simulink model "ex_hb1ode"  (R2023a)
settings: Solver=ode15s  StartTime=0.0  StopTime=1e5
undefined symbols (not defined in the file): k1, k2, k3
settings Model: Creator=mosuk  LastModifiedBy=mosuk
settings DataIOCC: ReturnWorkspaceOutputs=off

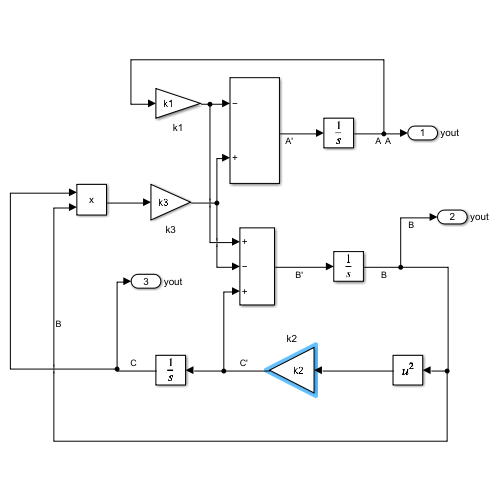
[thumbnail: Simulink's stored preview of the top-level diagram]
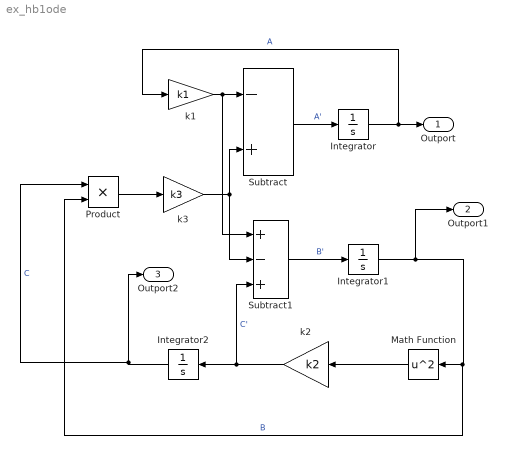
== system ex_hb1ode ==
  Integrator : Integrator  InitialCondition=1
  Integrator1 : Integrator
  Integrator2 : Integrator
  Math Function : Math  Operator=square
  Product : Product
  Subtract : Sum  Inputs=-+
  Subtract1 : Sum  Inputs=+-+
  k1 : Gain  Gain=k1
  k2 : Gain  Gain=k2
  k3 : Gain  Gain=k3
  Outport : Outport  SignalName=yout
  Outport1 : Outport  Port=2  SignalName=yout
  Outport2 : Outport  Port=3  SignalName=yout
  wires:
  k1/1 -> Subtract1/1, Subtract/1
  k3/1 -> Subtract1/2, Subtract/2
  Integrator/1 -> k1/1, Outport/1  "A"
  Subtract/1 -> Integrator/1  "A'"
  Product/1 -> k3/1
  Subtract1/1 -> Integrator1/1  "B'"
  Integrator1/1 -> Product/2, Math Function/1, Outport1/1  "B"
  Math Function/1 -> k2/1
  k2/1 -> Subtract1/3, Integrator2/1  "C'"
  Integrator2/1 -> Product/1, Outport2/1  "C"
